simulink model "sscv_wind_turbine"  (R2024a)
settings: Solver=ode23t  StartTime=0.0  StopTime=simT  RelTol=1e-3  AbsTol=1e-3
PreLoadFcn:
  | sscv_wind_turbine_input
values from neighbouring files (symbols this model uses):
  actuatorRampRate = 20    [sscv_wind_turbine_input.m]
  brakePressure = 100    [sscv_wind_turbine_input.m]
  controllerTimeConstant = 2    [sscv_wind_turbine_input.m]
  Derating = [12 13 14 15 16 17 18 19 20 1 4 7 ... (18 elements, 9x2)]    [sscv_wind_turbine_Derating.mat]
  generatorEfficiency = 90    [sscv_wind_turbine_input.m]
  generatorLumpedInductance = 1.9160e-04    (= 0.0001916)    [sscv_wind_turbine_input.m]
  generatorLumpedResistance = 0.0027    [sscv_wind_turbine_input.m]
  gridFrequency = 60    [sscv_wind_turbine_input.m]
  iGenerationGain = 1    [sscv_wind_turbine_input.m]
  maxPitchAngle = max(pitch)    [sscv_wind_turbine_input.m]
  minPitchAngle = min(pitch)    [sscv_wind_turbine_input.m]
  mpptOmega = [502.335 613.965 753.5025 865.1325 1004.67 1116.3 1200.0225 1200.0225 1200.0225]    [sscv_wind_turbine_MPPT.mat]
  mpptPower = [0.0596400180021 0.116487570967 0.201285060757 0.319665137738 0.477120144017 0.679427108153 0.931130687114 1.22525336077 1.55330342875]    [sscv_wind_turbine_MPPT.mat]
  mpptWindSpeed = [4 5 6 7 8 9 10 11 12]    [sscv_wind_turbine_MPPT.mat]
  pGenerationGain = 0.1    [sscv_wind_turbine_input.m]
  pGeneratorBrakeLimit = 0.50    (= 0.5)    [sscv_wind_turbine_input.m]
  pitchBrakeAngle = 95    [sscv_wind_turbine_input.m]
  turbineRatedPower = 1.5    [sscv_wind_turbine_input.m]
  vWindRated = 12    [sscv_wind_turbine_input.m]
  wAtGeneratorRatedPower = wTurbineCutOut*gearRatio    (= 1227.93)    [sscv_wind_turbine_input.m]
  wGeneratorBrakeLimit = 0.50    (= 0.5)    [sscv_wind_turbine_input.m]
undefined symbols (not defined in the file or in its folder): ee_sli_rtmsupport, G, gcbh
libraries: fl_lib x18, simulink x15, nesl_utility x13, ee_lib x10, sdl_lib x6, eeGeneralControl x3, eeGeneralMeasurement x2
(part 1 of 2)
CloseFcn:
  | try,close(h_sscv_wind_turbine),end
  | clear h_sscv_wind_turbine
  | 
  | clear airDensity cp pitch TSR turbineRadius
  | clear vWindThreshold wThreshold vWindCutInLower
  | clear vWindCutOut vWindCutInUpper vWindRated
  | clear wTurbineCutIn wTurbineCutOut wTurbinePark
  | clear pitchBrakeAngle minPitchAngle maxPitchAngle
  | clear actuatorRampRate controllerTimeConstant
  | clear turbineRatedPower pGenerationGain
  | clear brakePressure brakeTorqueRadius
  | clear brakePistonArea brakeStaticFrictionCoeff
  | clear brakeKineticFrictionCoeff brakeClutchVelocityTol
  | clear brakeThresholdPressure numFrictionSurfaces
  | clear rotorBladeInertia generatorInertia
  | clear carrierShaftInertia stepShaftInertia
  | clear ringSunTeethRatio firstStepTeethRatio
  | clear secondStepTeethRatio windProfile
  | clear Derating gearRatio
  | clear generatorEfficiency mpptOmega mpptPower
  | clear generatorLumpedInductance generatorLumpedResistance
  | clear gridFrequency iGenerationGain
  | clear mpptWindSpeed transformerPrimaryVoltage
  | clear transformerRatedPower transformerSecondaryVoltage
  | clear wGeneratorBrakeLimit wAtGeneratorRatedPower
  | clear cpBraking simT pGeneratorBrakeLimit
  | clear windProfile1 windProfile2 windProfile3
  | clear numTSR
  | clear logsout_sscv_wind_turbine
  | clear simlog_sscv_wind_turbine
Description:
  | Wind Turbine
settings Model: Creator=The MathWorks, Inc.  LastModifiedBy=The MathWorks, Inc.
settings SolverCC: AutoScaleAbsTol=off  MaxConsecutiveMinStep=5  AlgebraicLoopSolver=TrustRegion  MaxZcPerStep=1
settings DataIOCC: SaveOutput=off  DSMLogging=off  SaveTime=off  ReturnWorkspaceOutputs=off  SignalLoggingName=logsout_sscv_wind_turbine
settings OptimizationCC: ReuseModelBlockBuffer=off
settings DebuggingCC: UnconnectedInputMsg=warning  UnconnectedOutputMsg=warning  UnconnectedLineMsg=warning
settings ModelReferenceCC: EnableRefExpFcnMdlSchedulingChecks=on
settings RTWCC: GPUComputeCapability=3.5  DLArmComputeVersion=19.05
settings SimscapeCC: SimscapeLogType=all  SimscapeLogSimulationStatistics=on  SimscapeLogName=simlog_sscv_wind_turbine  SimscapeLogDataHistory=10000000

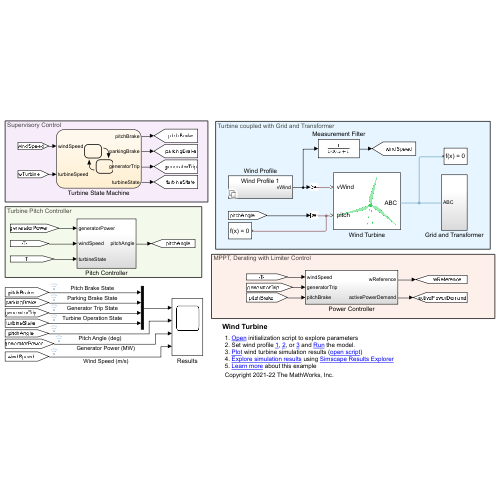
[thumbnail: Simulink's stored preview of the top-level diagram]
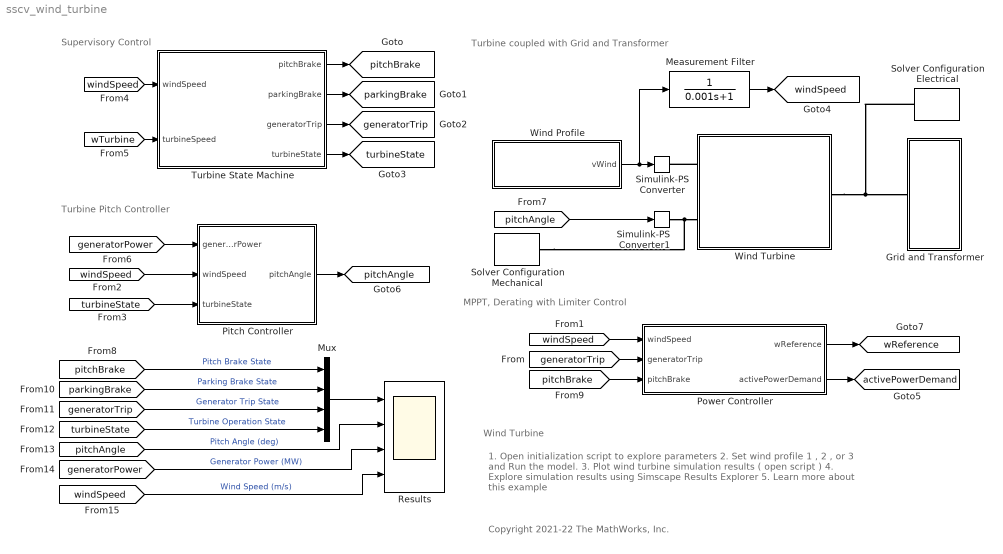
== system sscv_wind_turbine ==
  note: MPPT, Derating with Limiter Control
  note: Turbine coupled with Grid and Transformer
  note: Turbine Pitch Controller
  note: Supervisory Control
  note: 1. Open initialization script to explore parameters
      | 2. Set wind profile 1 , 2 , or 3 and Run the model.
      | 3. Plot wind turbine simulation results ( open script )
      | 4. Explore simulation results using Simscape Results Explorer
      | 5. Learn more about this example
  note: Wind Turbine
  note: Copyright 2021-22 The MathWorks, Inc.
  Grid and Transformer : Subsystem
  Measurement Filter : TransferFcn  Denominator=[0.001 1]
  Mux : Mux
  Pitch Controller : Subsystem
  Power Controller : Subsystem
  Results : Scope  NumInputPorts=4
  Simulink-PS Converter : nesl_utility/Simulink-PS Converter  PhysicalDomain=network_engine_domain  SubClassName=ps_input  LeftPortType=input  RightPortType=output  PseudoPeriodic=off  Frequencies=[]  NoiseDistribution=none  NoiseParameters=[]  Unit=m/s  AffineConversion=off  FilteringAndDerivatives=filter  SimscapeFilterOrder=1  InputFilterTimeConstant=0.001  UdotUserProvided=0
  Simulink-PS Converter1 : nesl_utility/Simulink-PS Converter  PhysicalDomain=network_engine_domain  SubClassName=ps_input  LeftPortType=input  RightPortType=output  PseudoPeriodic=off  Frequencies=[]  NoiseDistribution=none  NoiseParameters=[]  Unit=deg  AffineConversion=off  FilteringAndDerivatives=filter  SimscapeFilterOrder=1  InputFilterTimeConstant=0.001  UdotUserProvided=0
  Solver Configuration Electrical : nesl_utility/Solver Configuration  PhysicalDomain=network_engine_domain  SubClassName=solver  LeftPortType=input  RightPortType=generic  Tones=[]  Harmonics=[]  SimulateNoise=off  Profile=off  UseLocalSampling=off  EnableSwitchedLinearOptims=on  FrequencyDomain=off  UseCCode=off  RelTol=0.001  AbsTol=0.001  MinStep=1e-09  ToWorkspace=off  RevertToSquareIcSolve=off  NumHomotopyIterations=100  PhasorMode=off  PhasorModeNumHarmonics=1  ConsistencySolver=NEWTON_FTOL  IndexReductionMethod=DerivativeReplacement  DoDC=off  ResidualTolerance=1e-09  ConsistencyTolSource=GLOBAL  ConsistencyAbsTol=0.001  ConsistencyRelTol=0.001  ConsistencyTolFactor=0.001  UseLocalSolver=off  LocalSolverChoice=NE_TRAPEZOIDAL_ADVANCER  ResolveIndetEquations=on  FunctionEvalNumThread=1  LocalSolverSampleTime=1e-5  DoFixedCost=off  MaxNonlinIter=3  MaxModeIter=2  ComputeImpulses=off  ImpulseIterations=2  LinearAlgebra=auto  LinearAlgebraNumThread=0  EquationFormulation=NE_TIME_EF  DelaysMemoryBudget=1024  AutomaticFiltering=on  FilteringTimeConstant=0.001  PartitionStorageMethod=AS_NEEDED  PartitionMemoryBudget=1024  PartitionMethod=ROBUST  MultibodyUseLocalSolver=off  MultibodyLocalSolverChoice=ODE1  MultibodyLocalSolverSampleTime=0.001
  Solver Configuration Mechanical : nesl_utility/Solver Configuration  PhysicalDomain=network_engine_domain  SubClassName=solver  LeftPortType=input  RightPortType=generic  Tones=[]  Harmonics=[]  SimulateNoise=off  Profile=off  UseLocalSampling=off  EnableSwitchedLinearOptims=on  FrequencyDomain=off  UseCCode=off  RelTol=0.001  AbsTol=0.001  MinStep=1e-09  ToWorkspace=off  RevertToSquareIcSolve=off  NumHomotopyIterations=100  PhasorMode=off  PhasorModeNumHarmonics=1  ConsistencySolver=NEWTON_FTOL  IndexReductionMethod=DerivativeReplacement  DoDC=off  ResidualTolerance=1e-09  ConsistencyTolSource=GLOBAL  ConsistencyAbsTol=0.001  ConsistencyRelTol=0.001  ConsistencyTolFactor=0.001  UseLocalSolver=off  LocalSolverChoice=NE_TRAPEZOIDAL_ADVANCER  ResolveIndetEquations=on  FunctionEvalNumThread=1  LocalSolverSampleTime=0.001  DoFixedCost=off  MaxNonlinIter=3  MaxModeIter=2  ComputeImpulses=off  ImpulseIterations=2  LinearAlgebra=auto  LinearAlgebraNumThread=0  EquationFormulation=NE_TIME_EF  DelaysMemoryBudget=1024  AutomaticFiltering=on  FilteringTimeConstant=0.001  PartitionStorageMethod=AS_NEEDED  PartitionMemoryBudget=1024  PartitionMethod=ROBUST  MultibodyUseLocalSolver=off  MultibodyLocalSolverChoice=ODE1  MultibodyLocalSolverSampleTime=0.001
  Turbine State Machine : Stateflow chart  TreatAsAtomicUnit=on
  Wind Profile : Subsystem  Variant=on  VariantControl=Choice
  Wind Turbine : Subsystem
      mask Display:
      | image('sscv_wind_turbine.PNG');
      | port_label('LConn',1,' vWind')
      | port_label('LConn',2,' pitch')
      | port_label('RConn',1,'ABC ')
  tag scope: activePowerDemand=global, generatorTrip=global, parkingBrake=global, pitchAngle=global, pitchBrake=global, turbineState=global, wReference=global, windSpeed=global
  wires:
  Turbine State Machine/1(pitchBrake) -> [pitchBrake]
  Turbine State Machine/2(parkingBrake) -> [parkingBrake]
  Turbine State Machine/3(generatorTrip) -> [generatorTrip]
  Turbine State Machine/4(turbineState) -> [turbineState]
  [windSpeed] -> Turbine State Machine/1(windSpeed)
  [wTurbine] -> Turbine State Machine/2(turbineSpeed)
  [generatorPower] -> Pitch Controller/1(generatorPower)
  [turbineState] -> Pitch Controller/3(turbineState)
  [pitchAngle] -> Simulink-PS Converter1/1
  Measurement Filter/1 -> [windSpeed]
  [windSpeed] -> Power Controller/1(windSpeed)
  Power Controller/1(wReference) -> [wReference]
  Power Controller/2(activePowerDemand) -> [activePowerDemand]
  [generatorTrip] -> Power Controller/2(generatorTrip)
  Pitch Controller/1(pitchAngle) -> [pitchAngle]
  [windSpeed] -> Pitch Controller/2(windSpeed)
  [pitchBrake] -> Power Controller/3(pitchBrake)
  [pitchBrake] -> Mux/1  "Pitch Brake State"
  [parkingBrake] -> Mux/2  "Parking Brake State"
  [generatorTrip] -> Mux/3  "Generator Trip State"
  [turbineState] -> Mux/4  "Turbine Operation State"
  Mux/1 -> Results/1
  [pitchAngle] -> Results/2  "Pitch Angle (deg)"
  [generatorPower] -> Results/3  "Generator Power (MW)"
  [windSpeed] -> Results/4  "Wind Speed (m/s)"
  Wind Profile/1(vWind) -> Measurement Filter/1, Simulink-PS Converter/1
  connections:
  Wind Turbine/RConn1 -- Solver Configuration Electrical/RConn1 -- Grid and Transformer/LConn1
  Simulink-PS Converter1/RConn1 -- Solver Configuration Mechanical/RConn1 -- Wind Turbine/LConn2
  Wind Turbine/LConn1 -- Simulink-PS Converter/RConn1

== system sscv_wind_turbine/Grid and Transformer ==
  Electrical Reference : fl_lib/Electrical/Electrical Elements/Electrical Reference
  Grid : ee_lib/Sources/Voltage Source (Three-Phase)  vline_rms=transformerPrimaryVoltage kV  shift=0 deg  freq=gridFrequency Hz  impedance_option=0  SShortCircuit=1e6 A*V  XR=15  R=0.01 Ohm  L=3.97e-4 H  harmonic_option=0  harmonic_orders=[5, 7, 11, 13]  harmonic_ratios=[.1, .1, .1, .1]  G_parasitic=0 1/Ohm  I_specify=off  I_priority=None  I=[0, 0, 0] A  I_nominal_specify=off  I_nominal_value=1  I_nominal_unit=A
  Neutral Port (Three-Phase) : ee_lib/Connectors & References/Neutral Port (Three-Phase)  G_parasitic=1e-12 1/Ohm
      settings: InternalSimscapePortConfiguration="{\"Bottom\":[],\"Left\":[{\"id\":\"N\",\"label\":\"~\",\"type\":\"foundation.electrical.three_phase\"}],\"Right\":[{\"id\":\"n\",\"label\":\"n\",\"type\":\"foundation.electrical.electrical\"}],\"Top\":[]}"
  Parasitic Conductance : ee_lib/Passive/RLC Assemblies/RLC (Three-Phase)  component_structure=ee.enum.rlc.structure.R  R=100000 Ohm  L=1e-3 H  C=1e-6 F  R_parasitic=0 Ohm  G_parasitic=0 1/Ohm  IL_specify=off  IL_priority=High  IL=[0, 0, 0] A  IL_nominal_specify=off  IL_nominal_value=1  IL_nominal_unit=A  VC_specify=off  VC_priority=High  VC=[0, 0, 0] V  VC_nominal_specify=off  VC_nominal_value=1  VC_nominal_unit=V
      settings: InternalSimscapePortConfiguration="{\"Bottom\":[],\"Left\":[{\"id\":\"N1\",\"label\":\"~1\",\"type\":\"foundation.electrical.three_phase\"}],\"Right\":[{\"id\":\"N2\",\"label\":\"~2\",\"type\":\"foundation.electrical.three_phase\"}],\"Top\":[]}"
  Transformer : ee_lib/Passive/Transformers/Two-Winding Transformer (Three-Phase)  SRated=transformerRatedPower MW  FRated=gridFrequency Hz  Winding1Connection=ee.enum.windingconnection.Y  VRated1=transformerPrimaryVoltage kV  Winding2Connection=ee.enum.windingconnection.Y  VRated2=transformerSecondaryVoltage kV  CoreType=ee.enum.coretype.threelimb  pu_Rw1=0.0001  pu_Rw2=0.0001  leakage_reactance_option=ee.enum.transformer_leakage.exclude  pu_Xl1=0.05  pu_Xl2=0.05  magnetizing_resistance_option=ee.enum.transformer_magnetizingResistance.exclude  pu_Rm=500  magnetizing_reactance_option=ee.enum.transformer_magnetizingReactance.exclude  saturation_option=ee.enum.transformer_saturation.exclude  pu_Xm=500  current_data=[0, .002, 1, 2]  magnetic_flux_data=[0, 1.2, 1.5, 1.51]  pu_X0=0.5  i1_specify=off  i1_priority=None  i1=[0, 0, 0] A  i1_nominal_specify=off  i1_nominal_value=1  i1_nominal_unit=A  i2_specify=off  i2_priority=None  i2=[0, 0, 0] A  i2_nominal_specify=off  i2_nominal_value=1  i2_nominal_unit=A  phi_specify=off  phi_priority=None  phi=[0, 0, 0]  phi_nominal_specify=off  phi_nominal_value=1  phi_nominal_unit=1  power_dissipated_specify=off  power_dissipated_priority=None  power_dissipated=0 W  power_dissipated_nominal_specify=off  power_dissipated_nominal_value=1  power_dissipated_nominal_unit=W
      settings: InternalSimscapePortConfiguration="{\"Bottom\":[],\"Left\":[{\"id\":\"N1\",\"label\":\"~1\",\"type\":\"foundation.electrical.three_phase\"}],\"Right\":[{\"id\":\"N2\",\"label\":\"~2\",\"type\":\"foundation.electrical.three_phase\"}],\"Top\":[]}"
  ABC : PMIOPort  Side=Left
  connections:
  Transformer/RConn1 -- Parasitic Conductance/LConn1 -- ABC/RConn1
  Neutral Port (Three-Phase)/RConn1 -- Electrical Reference/LConn1 -- Grid/LConn1
  Neutral Port (Three-Phase)/LConn1 -- Parasitic Conductance/RConn1
  Transformer/LConn1 -- Grid/RConn1

== system sscv_wind_turbine/Pitch Controller ==
  generatorPower : Inport
  windSpeed : Inport  Port=2
  turbineState : Inport  Port=3
  Merge : Merge  Inputs=3
  Pitch Change Rate Limiter : RateLimiter  RisingSlewLimit=actuatorRampRate  FallingSlewLimit=-actuatorRampRate  SampleTimeMode=inherited
  Transfer Fcn1 : TransferFcn  Denominator=[1e-4 1]
  "Turbine State 0 : Park Brake and Turbine State 3 : Pitch Brake" : Subsystem
      settings: PortSchema="{\"entries\":[{\"content\":{\"sides\":[{\"content\":{\"connectorIds\":[\"In1\"]},\"type\":\"ConnectorPlacement.EquallySpacedRectSide\",\"uuid\":\"c81c0fc4-0b31-4a43-acf3-ef02f67f12ef\"},{\"content\":{\"connectorIds\":[\"In2\",\"Out1\"],\"side\":\"RIGHT\"},\"type\":\"ConnectorPlacement.EquallySpacedRectSide\",\"uuid\":\"c20c9bc8-a4c7-4c6f-a8fa-fe8ff88298f7\"},{\"content\":{\"connectorIds\":[],\"side\":\"TOP\"},\"type\":\"ConnectorPlacement.EquallySpacedRectSide\",\"uuid\":\"2b845051-401f-423c-a453-0a1243a015d1\"}]},\"type\":\"ConnectorPlacement.EquallySpacedConnector\",\"uuid\":\"502647d6-ee95-4637-92b5-6d3c38784edf\"}],\"packageUris\":[\"http://schema.mathworks.com/mf0/Connector/R2020b\"],\"version\":\"1.0\"}"
  "Turbine State 1 : Startup Condition" : Subsystem
  "Turbine State 2 : Power Generation Condition" : Subsystem
  pitchAngle : Outport
  wires:
  Pitch Change Rate Limiter/1 -> pitchAngle/1
  turbineState/1 -> "Turbine State 2 : Power Generation Condition"/3(turbineState), "Turbine State 0 : Park Brake and Turbine State 3 : Pitch Brake"/1(turbineState), "Turbine State 1 : Startup Condition"/1(turbineState)
  generatorPower/1 -> "Turbine State 2 : Power Generation Condition"/1(generatorPower)
  Merge/1 -> Pitch Change Rate Limiter/1, Transfer Fcn1/1
  "Turbine State 0 : Park Brake and Turbine State 3 : Pitch Brake"/1(pitchAngle) -> Merge/1
  "Turbine State 1 : Startup Condition"/1(pitchAngle) -> Merge/2
  "Turbine State 2 : Power Generation Condition"/1(pitchAngle) -> Merge/3
  windSpeed/1 -> "Turbine State 2 : Power Generation Condition"/2(windSpeed)
  Transfer Fcn1/1 -> "Turbine State 0 : Park Brake and Turbine State 3 : Pitch Brake"/2(pitchState)

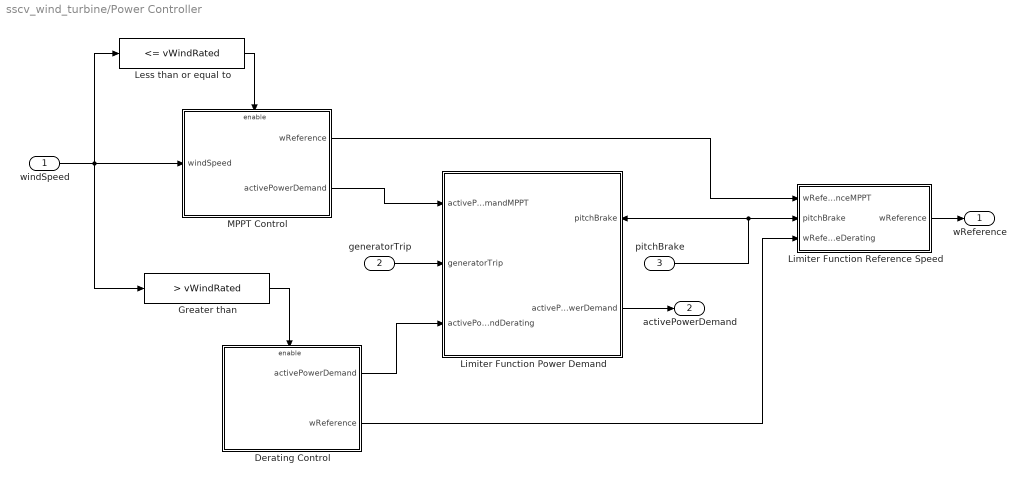
== system sscv_wind_turbine/Power Controller ==
  windSpeed : Inport
  generatorTrip : Inport  Port=2
  pitchBrake : Inport  Port=3
  Derating Control : Subsystem
  Greater than : simulink/Logic and Bit Operations/Compare To Constant  relop=>  const=vWindRated  OutDataTypeStr=boolean
  Less than or equal to : simulink/Logic and Bit Operations/Compare To Constant  relop=<=  const=vWindRated  OutDataTypeStr=boolean
  Limiter Function Power Demand : Subsystem
      settings: PortSchema="{\"entries\":[{\"content\":{\"sides\":[{\"content\":{\"connectorIds\":[\"In1\",\"In2\",\"In3\"]},\"type\":\"ConnectorPlacement.EquallySpacedRectSide\",\"uuid\":\"b03cf57d-370b-4fa1-bd93-9b836e03697e\"},{\"content\":{\"connectorIds\":[\"In4\",\"Out1\"],\"side\":\"RIGHT\"},\"type\":\"ConnectorPlacement.EquallySpacedRectSide\",\"uuid\":\"152758c3-43df-447a-a50f-afca466b3eeb\"},{\"content\":{\"connectorIds\":[],\"side\":\"TOP\"},\"type\":\"ConnectorPlacement.EquallySpacedRectSide\",\"uuid\":\"d053be3f-8f1f-4fa1-8d53-3d41a1fdecc7\"}]},\"type\":\"ConnectorPlacement.EquallySpacedConnector\",\"uuid\":\"ad588a80-a06e-49b6-a4d2-a4be271ff49a\"}],\"packageUris\":[\"http://schema.mathworks.com/mf0/Connector/R2020b\"],\"version\":\"1.0\"}"
  Limiter Function Reference Speed : Subsystem
  MPPT Control : Subsystem
  wReference : Outport
  activePowerDemand : Outport  Port=2
  wires:
  windSpeed/1 -> Greater than/1, Less than or equal to/1, MPPT Control/1(windSpeed)
  Less than or equal to/1 -> MPPT Control/Enable
  Greater than/1 -> Derating Control/Enable
  MPPT Control/2(activePowerDemand) -> Limiter Function Power Demand/1(activePowerDemandMPPT)
  generatorTrip/1 -> Limiter Function Power Demand/2(generatorTrip)
  Derating Control/1(activePowerDemand) -> Limiter Function Power Demand/3(activePowerDemandDerating)
  Limiter Function Power Demand/1(activePowerDemand) -> activePowerDemand/1
  pitchBrake/1 -> Limiter Function Reference Speed/2(pitchBrake), Limiter Function Power Demand/4(pitchBrake)
  MPPT Control/1(wReference) -> Limiter Function Reference Speed/1(wReferenceMPPT)
  Derating Control/2(wReference) -> Limiter Function Reference Speed/3(wReferenceDerating)
  Limiter Function Reference Speed/1(wReference) -> wReference/1

== system sscv_wind_turbine/Wind Profile ==
  Wind Profile 1 : Subsystem  VariantControl=windProfile1
  Wind Profile 2 : Subsystem  VariantControl=windProfile2
  Wind Profile 3 : Subsystem  VariantControl=windProfile3
  vWind : Outport

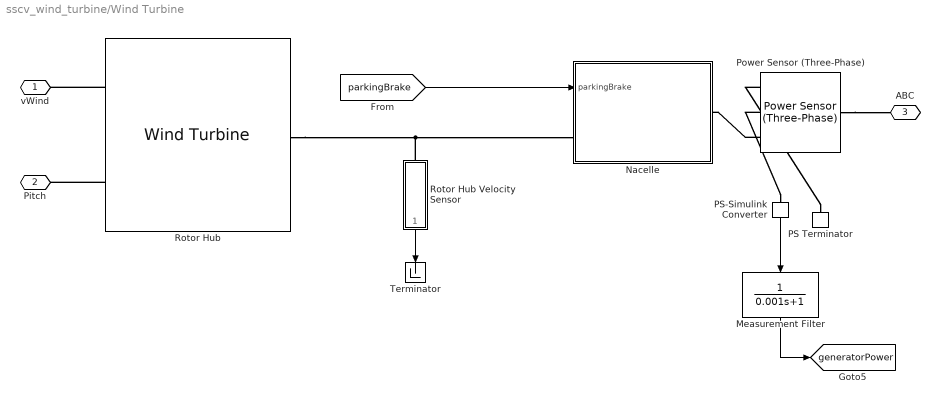
== system sscv_wind_turbine/Wind Turbine ==
  Measurement Filter : TransferFcn  Denominator=[0.001 1]
  Nacelle : Subsystem
  PS Terminator : fl_lib/Physical Signals/Sinks/PS Terminator
  PS-Simulink Converter : nesl_utility/PS-Simulink Converter  PhysicalDomain=network_engine_domain  SubClassName=ps_output  LeftPortType=input  RightPortType=output  PseudoPeriodic=off  Frequencies=[]  VectorFormat=inherit  Unit=MW  AffineConversion=off
  Power Sensor (Three-Phase) : ee_lib/Sensors & Transducers/Power Sensor (Three-Phase)  load_type=ee.enum.passive.type_balanced.balanced  f0=60 Hz  config=ee.enum.with_neutral.no  rho=1
      settings: InternalSimscapePortConfiguration="{\"Bottom\":[],\"Left\":[{\"id\":\"N1\",\"label\":\"~1\",\"type\":\"foundation.electrical.three_phase\"}],\"Right\":[{\"id\":\"N2\",\"label\":\"~2\",\"type\":\"foundation.electrical.three_phase\"}],\"Top\":[{\"id\":\"Pm\",\"label\":\"P\",\"type\":\"output\"},{\"id\":\"Qm\",\"label\":\"Q\",\"type\":\"output\"}]}"
  Rotor Hub : sdl_lib/Engines & Motors/Wind Turbine  parameterization=sdl.enum.WindTurbineParameterization.PowerThrust  R_rotor=turbineRadius m  pitch_TLU=pitch deg  lambda_TLU=TSR  Cp_TLU=cp  Ct_TLU=[0.0777, 0.1421, 0.3753, 0.6599, 0.8160, 0.9112, 0.9925, 1.0708, 1.1147; 0.0762, 0.1377, 0.3570, 0.5529, 0.6291, 0.6573, 0.6706, 0.6421, 0.6284; 0.0682, 0.1292, 0.3362, 0.4664, 0.4874, 0.4547, 0.3915, 0.2865, 0.2249; -0.05 * ones(1, 9)]  n_blades=3  radial_TLU=[.1, .17, .23, .36, .5, .63, 1]  twist_TLU=[13.31, 13.31, 11.48, 9.01, 6.54, 4.19, .11] deg  chord_TLU=[.068, .074, .076, .069, .061, .053, .023]  alpha_TLU=[-180 : 10 : 180] deg  Cl_TLU=[0, 0, 0, 0, 0, 0, 0; 0, .397, .547, .547, .735, .788, .749; 0, .642, .685, .685, .695, .67, .659; 0, .757, .816, .816, .828, .797, .783; 0, .762, .832, .832, .846, .813, .798; 0, .68, .756, .756, .771, .739, .724; 0, .532, .609, .609, .624, .596, .581; 0, .337, .411, .411, .426, .403, .39; 0, .114, .182, .182, .195, .179, .169; 0, -.12, -.061, -.061, -.05, -.06, -.067; 0, -.349, -.302, -.302, -.294, -.295, -.299; 0, -.557, -.523, -.523, -.518, -.512, -.512; 0, -.727, -.708, -.708, -.706, -.693, -.689; 0, -.842, -.838, -.838, -.839, -.82, -.814; 0, -.886, -.895, -.895, -.898, -.875, -.866; 0, -.839, -.858, -.858, -.862, -.838, -.829; 0, -.685, -1.013, -1.013, -.815, -.869, -.958; 0, -.311, -.8496, -.8496, -.8284, -.8284, -.711; 0, .137, .288, .288, .444, .521, .442; 0, 1.368, 1.458, 1.458, 1.442, 1.358, 1.382; 0, 1.7825, 1.398, 1.398, 1.354, 1.311, 1.428; 0, 1.904, 1.265, 1.265, 1.076, .962, .926; 0, 1.903, 1.258, 1.258, 1.064, .95, .804; 0, 1.69, 1.146, 1.146, .98, .884, .763; 0, 1.323, .932, .932, .81, .74, .656; 0, .88, .657, .657, .582, .54, .495; 0, .449, .362, .362, .326, .304, .291; 0, .124, .092, .092, .072, .053, .053; 0, -.118, -.15, -.15, -.17, -.198, -.199; 0, -.348, -.379, -.379, -.399, -.434, -.436; 0, -.549, -.578, -.578, -.596, -.637, -.64; 0, -.702, -.727, -.727, -.743, -.787, -.79; 0, -.787, -.807, -.807, -.821, -.864, -.868; 0, -.782, -.797, -.797, -.806, -.847, -.85; 0, -.664, -.673, -.673, -.679, -.711, -.714; 0, -.41, -.547, -.547, -.735, -.788, -.749; 0, 0, 0, 0, 0, 0, 0]  Cd_TLU=[.35, .0602, .0267, .0267, .0202, .0185, .0198; .35, .1107, .0968, .0968, .0943, .0945, .0955; .35, .3045, .2876, .2876, .2848, .2809, .2807; .35, .5355, .5232, .5232, .5215, .5112, .5086; .35, .7685, .7656, .7656, .766, .7485, .7427; .35, .9788, .9882, .9882, .9911, .9665, .9574; .35, 1.1499, 1.173, 1.173, 1.1787, 1.1476, 1.1355; .35, 1.2716, 1.3084, 1.3084, 1.3168, 1.2805, 1.2656; .35, 1.3378, 1.3875, 1.3875, 1.3984, 1.3582, 1.341; .35, 1.346, 1.407, 1.407, 1.4201, 1.3774, 1.3587; .35, 1.2964, 1.3664, 1.3664, 1.3811, 1.3376, 1.3181; .35, 1.1918, 1.2676, 1.2676, 1.2833, 1.2409, 1.2212; .35, 1.0376, 1.1156, 1.1156, 1.1315, 1.0919, 1.0731; .35, .8429, .9187, .9187, .9341, .899, .882; .35, .6215, .6904, .6904, .7042, .6754, .661; .35, .3932, .4503, .4503, .4616, .4405, .4295; .35, .1861, .2388, .2388, .2237, .1983, .1785; .35, .0931, .0718, .0718, .0287, .0287, .0111; .35, .0113, .0087, .0087, .0065, .0057, .0052; .35, .0393, .0192, .0192, .0262, .0255, .015; .35, .3998, .2689, .2689, .228, .1987, .2379; .35, .8441, .5843, .5843, .5149, .4813, .4294; .35, 1.2873, .897, .897, .7901, .7396, .6452; .35, 1.6401, 1.1686, 1.1686, 1.0378, .9781, .8664; .35, 1.836, 1.3647, 1.3647, 1.2333, 1.1796, 1.0693; .35, 1.8347, 1.4621, 1.4621, 1.3587, 1.3297, 1.2438; .35, 1.6334, 1.4544, 1.4544, 1.4063, 1.4202, 1.3809; .35, 1.3879, 1.3938, 1.3938, 1.3985, 1.4512, 1.4565; .35, 1.3795, 1.3798, 1.3798, 1.381, 1.4294, 1.4345; .35, 1.3114, 1.3063, 1.3063, 1.3041, 1.3464, 1.3512; .35, 1.1864, 1.1763, 1.1763, 1.1709, 1.2057, 1.2099; .35, 1.0102, .9962, .9962, .9883, 1.0144, 1.0179; .35, .7935, .7771, .7771, .7676, .7845, .7871; .35, .5532, .5364, .5364, .5264, .5346, .5363; .35, .3147, .3, .3, .2912, .2922, .2931; .35, .1144, .1051, .1051, .0995, .0969, .0971; .35, .0602, .0267, .0267, .0202, .0185, .0198]  n_blade_discretization=20  model_thrust=false  model_inertia=sdl.enum.model_inertia.on  rotor_inertia=rotorBladeInertia kg*m^2  init_rot_vel=0 rad/s  rho_air=airDensity kg/m^3  v_thr=0.01 m/s  w_thr=0.01 rad/s  root_pitch=0 deg  expose_port_C=0
      settings: InternalSimscapePortConfiguration="{\"Bottom\":[],\"Left\":[{\"id\":\"vWind\",\"label\":\"V\",\"type\":\"input\"},{\"id\":\"pitch\",\"label\":\"β\",\"type\":\"input\"}],\"Right\":[{\"id\":\"R\",\"label\":\"R\",\"type\":\"foundation.mechanical.rotational.rotational\"}],\"Top\":[]}"
  Rotor Hub Velocity Sensor : Subsystem
  Terminator : Terminator
  vWind : PMIOPort  Side=Left
  Pitch : PMIOPort  Port=2  Side=Left
  ABC : PMIOPort  Port=3  Side=Right
  tag scope: generatorPower=global
  wires:
  Rotor Hub Velocity Sensor/1(wTurbine) -> Terminator/1
  [parkingBrake] -> Nacelle/1(parkingBrake)
  PS-Simulink Converter/1 -> Measurement Filter/1
  Measurement Filter/1 -> [generatorPower]
  connections:
  Rotor Hub/LConn1 -- vWind/RConn1
  Rotor Hub/LConn2 -- Pitch/RConn1
  Rotor Hub Velocity Sensor/LConn1 -- Rotor Hub/RConn1 -- Nacelle/LConn1
  Power Sensor (Three-Phase)/RConn1 -- ABC/RConn1
  Power Sensor (Three-Phase)/LConn1 -- Nacelle/RConn1
  Power Sensor (Three-Phase)/LConn2 -- PS-Simulink Converter/LConn1
  Power Sensor (Three-Phase)/LConn3 -- PS Terminator/LConn1

== system sscv_wind_turbine/Pitch Controller/Turbine State 0 : Park Brake and Turbine State 3 : Pitch Brake ==
  turbineState : Inport
  pitchState : Inport  Port=2
  Compare To Constant : simulink/Logic and Bit Operations/Compare To Constant  relop===  const=0  OutDataTypeStr=boolean
  Compare To Constant1 : simulink/Logic and Bit Operations/Compare To Constant  relop===  const=3  OutDataTypeStr=boolean
  OR : Logic  Operator=OR  IconShape=distinctive  AllPortsSameDT=off  OutDataTypeStr=boolean
  Turbine State 0 an 3 : Subsystem
  pitchAngle : Outport
  wires:
  Turbine State 0 an 3/1(pitchAngle) -> pitchAngle/1
  turbineState/1 -> Compare To Constant1/1, Compare To Constant/1
  pitchState/1 -> Turbine State 0 an 3/1(pitchState)
  OR/1 -> Turbine State 0 an 3/Enable
  Compare To Constant/1 -> OR/1
  Compare To Constant1/1 -> OR/2

== system sscv_wind_turbine/Pitch Controller/Turbine State 1 : Startup Condition ==
  turbineState : Inport
  Compare To Constant : simulink/Logic and Bit Operations/Compare To Constant  relop===  const=1  OutDataTypeStr=boolean
  Turbine State 1 : Subsystem
  pitchAngle : Outport
  wires:
  turbineState/1 -> Compare To Constant/1
  Compare To Constant/1 -> Turbine State 1/Enable
  Turbine State 1/1(pitchAngle) -> pitchAngle/1

== system sscv_wind_turbine/Pitch Controller/Turbine State 2 : Power Generation Condition ==
  generatorPower : Inport
  windSpeed : Inport  Port=2
  turbineState : Inport  Port=3
  Compare To Constant : simulink/Logic and Bit Operations/Compare To Constant  relop===  const=2  OutDataTypeStr=boolean
  Turbine State 2 : Subsystem
  pitchAngle : Outport
  wires:
  Turbine State 2/1(pitchAngle) -> pitchAngle/1
  Compare To Constant/1 -> Turbine State 2/Enable
  turbineState/1 -> Compare To Constant/1
  generatorPower/1 -> Turbine State 2/1(generatorPower)
  windSpeed/1 -> Turbine State 2/2(windSpeed)

== system sscv_wind_turbine/Power Controller/Derating Control ==
  Enable : EnablePort  StatesWhenEnabling=reset
  Constant : Constant  Value=turbineRatedPower
  Constant1 : Constant  Value=wAtGeneratorRatedPower
  Gain : Gain  Gain=100/generatorEfficiency
  MW to W : Gain  Gain=1e6
  activePowerDemand : Outport
  wReference : Outport  Port=2
  wires:
  Constant1/1 -> wReference/1
  MW to W/1 -> activePowerDemand/1
  Constant/1 -> Gain/1
  Gain/1 -> MW to W/1

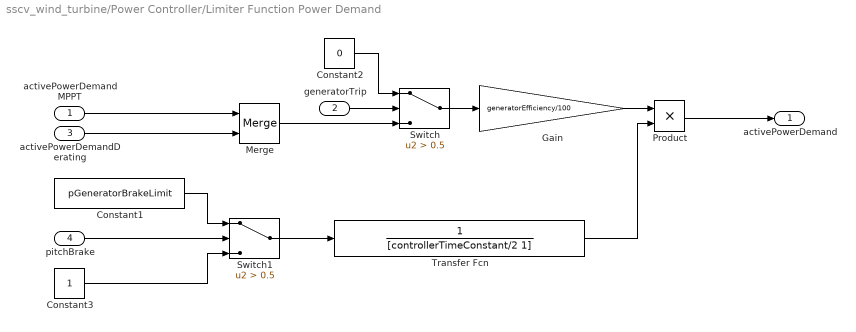
== system sscv_wind_turbine/Power Controller/Limiter Function Power Demand ==
  activePowerDemandMPPT : Inport
  generatorTrip : Inport  Port=2
  activePowerDemandDerating : Inport  Port=3
  pitchBrake : Inport  Port=4
  Constant1 : Constant  Value=pGeneratorBrakeLimit
  Constant2 : Constant  Value=0
  Constant3 : Constant
  Gain : Gain  Gain=generatorEfficiency/100
  Merge : Merge
  Product : Product
  Switch : Switch  Criteria=u2 > Threshold  Threshold=0.5  SaturateOnIntegerOverflow=off  InputSameDT=off
  Switch1 : Switch  Criteria=u2 > Threshold  Threshold=0.5  SaturateOnIntegerOverflow=off  InputSameDT=off
  Transfer Fcn : TransferFcn  Denominator=[controllerTimeConstant/2 1]
  activePowerDemand : Outport
  wires:
  generatorTrip/1 -> Switch/2
  Switch/1 -> Gain/1
  Constant2/1 -> Switch/1
  Merge/1 -> Switch/3
  activePowerDemandMPPT/1 -> Merge/1
  activePowerDemandDerating/1 -> Merge/2
  pitchBrake/1 -> Switch1/2
  Constant3/1 -> Switch1/3
  Constant1/1 -> Switch1/1
  Gain/1 -> Product/1
  Switch1/1 -> Transfer Fcn/1
  Product/1 -> activePowerDemand/1
  Transfer Fcn/1 -> Product/2

== system sscv_wind_turbine/Power Controller/Limiter Function Reference Speed ==
  wReferenceMPPT : Inport
  pitchBrake : Inport  Port=2
  wReferenceDerating : Inport  Port=3
  Constant : Constant
  Constant1 : Constant  Value=wGeneratorBrakeLimit
  Merge1 : Merge
  Product : Product
  Switch1 : Switch  Criteria=u2 > Threshold  Threshold=0.5  SaturateOnIntegerOverflow=off  InputSameDT=off
  Transfer Fcn : TransferFcn  Denominator=[controllerTimeConstant/2 1]
  wReference : Outport
  wires:
  pitchBrake/1 -> Switch1/2
  Constant1/1 -> Switch1/1
  wReferenceMPPT/1 -> Merge1/1
  wReferenceDerating/1 -> Merge1/2
  Merge1/1 -> Product/2
  Constant/1 -> Switch1/3
  Product/1 -> wReference/1
  Transfer Fcn/1 -> Product/1
  Switch1/1 -> Transfer Fcn/1

== system sscv_wind_turbine/Power Controller/MPPT Control ==
  windSpeed : Inport
  Enable : EnablePort  StatesWhenEnabling=reset
  MW to W : Gain  Gain=1e6
  mpptActivePowerDemand : Lookup_n-D  NumberOfTableDimensions=1  BreakpointsForDimension1=mpptWindSpeed  Table=mpptPower  InternalRulePriority=Speed  RndMeth=Simplest
  mpptOmega : Lookup_n-D  NumberOfTableDimensions=1  BreakpointsForDimension1=mpptWindSpeed  Table=mpptOmega  InternalRulePriority=Speed  RndMeth=Simplest
  wReference : Outport
  activePowerDemand : Outport  Port=2
  wires:
  mpptActivePowerDemand/1 -> MW to W/1
  mpptOmega/1 -> wReference/1
  windSpeed/1 -> mpptActivePowerDemand/1, mpptOmega/1
  MW to W/1 -> activePowerDemand/1

== system sscv_wind_turbine/Wind Profile/Wind Profile 1 ==
  Ramp : simulink/Sources/Ramp  slope=1  start=45  InitialOutput=15
  Saturation : Saturate  UpperLimit=22  LowerLimit=0
  vWind : Outport
  wires:
  Ramp/1 -> Saturation/1
  Saturation/1 -> vWind/1

== system sscv_wind_turbine/Wind Profile/Wind Profile 2 ==
  Add : Sum  Inputs=+
  Mux : Mux  Inputs=3
  Ramp : simulink/Sources/Ramp  slope=0.7  start=0  InitialOutput=0
  Ramp1 : simulink/Sources/Ramp  slope=0.7  start=115  InitialOutput=0
  Ramp2 : simulink/Sources/Ramp  slope=-0.7  start=160  InitialOutput=0
  Saturation : Saturate  UpperLimit=10  LowerLimit=0
  Saturation1 : Saturate  UpperLimit=12  LowerLimit=0
  Saturation2 : Saturate  UpperLimit=0  LowerLimit=-7
  vWind : Outport
  wires:
  Saturation1/1 -> Mux/2
  Ramp/1 -> Saturation/1
  Ramp2/1 -> Saturation2/1
  Add/1 -> vWind/1
  Saturation/1 -> Mux/1
  Ramp1/1 -> Saturation1/1
  Mux/1 -> Add/1
  Saturation2/1 -> Mux/3

== system sscv_wind_turbine/Wind Profile/Wind Profile 3 ==
  Ramp : simulink/Sources/Ramp  slope=1  start=45  InitialOutput=15
  Saturation : Saturate  UpperLimit=17  LowerLimit=0
  vWind : Outport
  wires:
  Ramp/1 -> Saturation/1
  Saturation/1 -> vWind/1

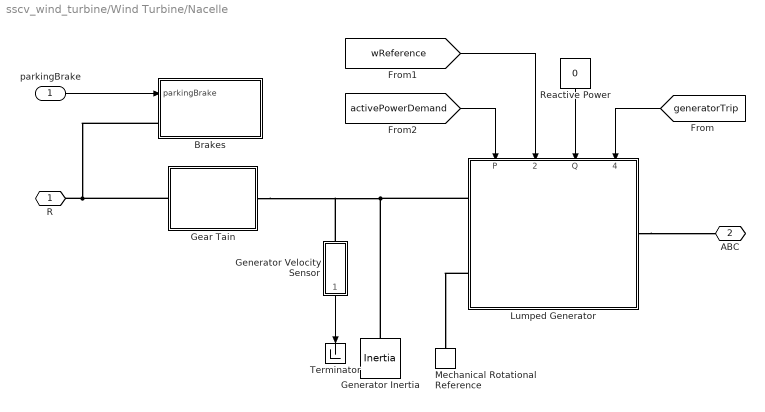
== system sscv_wind_turbine/Wind Turbine/Nacelle ==
  parkingBrake : Inport
  Brakes : Subsystem
  Gear Tain : Subsystem
  Generator Inertia : fl_lib/Mechanical/Rotational Elements/Inertia  inertia=generatorInertia kg*m^2  num_ports=foundation.enum.numPorts2.one  w_specify=on  w_priority=None  w=0 rad/s  w_nominal_specify=off  w_nominal_value=1  w_nominal_unit=rad/s  t_specify=off  t_priority=None  t=0 N*m  t_nominal_specify=off  t_nominal_value=1  t_nominal_unit=N*m
  "Generator Velocity Sensor " : Subsystem
  Lumped Generator : Subsystem  mask{ratedPower=turbineRatedPower, gridFreq=gridFrequency, genResistor=generatorLumpedResistance, genInductance=generatorLumpedInductance, genEfficiency=generatorEfficiency, ratedSpeed=wAtGeneratorRatedPower}
      mask prompts: ratedPower "Rated power (MW)"; gridFreq "Grid frequency (Hz)"; genResistor "Electrical generator lumped resistance (Ohm)"; genInductance "Electrical generator lumped leakage inductance (H)"; genEfficiency "Electrical generator effficiency"; ratedSpeed "Wind turbine speed at rated wind speed (rpm)"
      settings: PortSchema="{\"entries\":[{\"content\":{\"sides\":[{\"content\":{\"connectorIds\":[\"LConn1\",\"LConn2\"]},\"type\":\"ConnectorPlacement.EquallySpacedRectSide\",\"uuid\":\"600b86f2-4f8f-493b-ad26-1faa8bb85470\"},{\"content\":{\"connectorIds\":[\"RConn1\"],\"side\":\"RIGHT\"},\"type\":\"ConnectorPlacement.EquallySpacedRectSide\",\"uuid\":\"9e1649b7-9973-42e8-ab8f-93eff55c3d74\"},{\"content\":{\"connectorIds\":[\"In1\",\"In2\",\"In3\",\"In4\"],\"side\":\"TOP\"},\"type\":\"ConnectorPlacement.EquallySpacedRectSide\",\"uuid\":\"66dc1112-3744-4fa2-a344-a6dc92e314fc\"},{\"content\":{\"connectorIds\":[],\"side\":\"BOTTOM\"},\"type\":\"ConnectorPlacement.EquallySpacedRectSide\",\"uuid\":\"0ba4da35-be81-423d-9ede-c806323f0c4b\"}]},\"type\":\"ConnectorPlacement.EquallySpacedConnector\",\"uuid\":\"3b2d2e6e-f4ee-4b4b-84c0-3ef19b29de27\"}],\"packageUris\":[\"http://schema.mathworks.com/mf0/Connector/R2020b\"],\"version\":\"1.0\"}"
      mask Display: disp('Lumped Generator');
  Mechanical Rotational Reference : fl_lib/Mechanical/Rotational Elements/Mechanical Rotational Reference
  Reactive Power : Constant  Value=0
  Terminator : Terminator
  R : PMIOPort  Side=Left
  ABC : PMIOPort  Port=2  Side=Right
  wires:
  "Generator Velocity Sensor "/1(wGen) -> Terminator/1
  parkingBrake/1 -> Brakes/1(parkingBrake)
  [wReference] -> Lumped Generator/2(rotorSpeed)
  Reactive Power/1 -> Lumped Generator/3(Q)
  [activePowerDemand] -> Lumped Generator/1(P)
  [generatorTrip] -> Lumped Generator/4(generatorTrip)
  connections:
  Lumped Generator/LConn2 -- Mechanical Rotational Reference/LConn1
  Gear Tain/LConn1 -- Brakes/LConn1 -- R/RConn1
  Generator Inertia/LConn1 -- Lumped Generator/LConn1 -- Gear Tain/RConn1 -- "Generator Velocity Sensor "/LConn1
  Lumped Generator/RConn1 -- ABC/RConn1

== system sscv_wind_turbine/Wind Turbine/Rotor Hub Velocity Sensor ==
  Ideal Rotational Motion Sensor : fl_lib/Mechanical/Mechanical Sensors/Ideal Rotational Motion Sensor  reference=foundation.enum.MeasurementReference.difference  acceleration_port=false  velocity_port=true  position_port=true  wrap_angle=simscape.enum.onoff.off  offset=0 rad
  Measurement Filter : TransferFcn  Denominator=[0.001 1]
  Mechanical Rotational Reference2 : fl_lib/Mechanical/Rotational Elements/Mechanical Rotational Reference
  PS-Simulink Converter : nesl_utility/PS-Simulink Converter  PhysicalDomain=network_engine_domain  SubClassName=ps_output  LeftPortType=input  RightPortType=output  PseudoPeriodic=off  Frequencies=[]  VectorFormat=1-D array  Unit=rpm  AffineConversion=off
  R : PMIOPort  Side=Left
  wTurbine : Outport
  tag scope: wTurbine=global
  wires:
  PS-Simulink Converter/1 -> Measurement Filter/1
  Measurement Filter/1 -> [wTurbine], wTurbine/1
  connections:
  Ideal Rotational Motion Sensor/RConn2 -- PS-Simulink Converter/LConn1
  Ideal Rotational Motion Sensor/LConn1 -- R/RConn1
  Ideal Rotational Motion Sensor/RConn1 -- Mechanical Rotational Reference2/LConn1

== system sscv_wind_turbine/Pitch Controller/Turbine State 0 : Park Brake and Turbine State 3 : Pitch Brake/Turbine State 0 an 3 ==
  note: Turbine State 0 & 3: Park & Pitch Brake
  pitchState : Inport
  Enable : EnablePort  StatesWhenEnabling=reset
  Constant : Constant  Value=pitchBrakeAngle
  Constant1 : Constant
  Controller : TransferFcn  Denominator="[controllerTimeConstant  1]"
  Integrator : Integrator
  Switch : Switch  Criteria=u2 > Threshold  Threshold=controllerTimeConstant*log(1-(maxPitchAngle/pitchBrakeAngle))*(-1.01)  SaturateOnIntegerOverflow=off  InputSameDT=off
  pitchAngle : Outport
  wires:
  Integrator/1 -> Switch/2
  pitchState/1 -> Switch/3
  Constant1/1 -> Integrator/1
  Constant/1 -> Controller/1
  Controller/1 -> Switch/1
  Switch/1 -> pitchAngle/1

== system sscv_wind_turbine/Pitch Controller/Turbine State 1 : Startup Condition/Turbine State 1 ==
  note: Turbine State 1: Startup
  Enable : EnablePort  StatesWhenEnabling=reset
  Constant : Constant  Value=minPitchAngle
  Saturation : Saturate  UpperLimit=maxPitchAngle  LowerLimit=minPitchAngle
  Transfer Fcn : TransferFcn  Denominator=[controllerTimeConstant 1]
  pitchAngle : Outport
  wires:
  Constant/1 -> Transfer Fcn/1
  Saturation/1 -> pitchAngle/1
  Transfer Fcn/1 -> Saturation/1

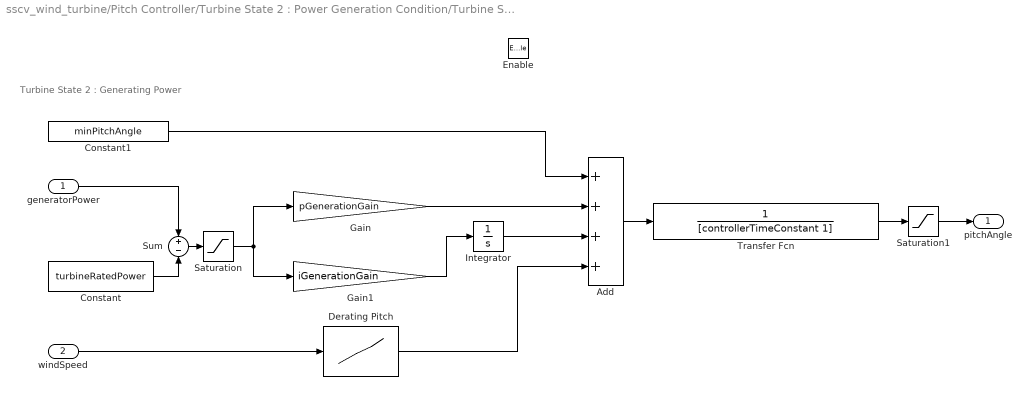
== system sscv_wind_turbine/Pitch Controller/Turbine State 2 : Power Generation Condition/Turbine State 2 ==
  note: Turbine State 2 : Generating Power
  generatorPower : Inport
  windSpeed : Inport  Port=2
  Enable : EnablePort  StatesWhenEnabling=reset
  Add : Sum  Inputs=++++
  Constant : Constant  Value=turbineRatedPower
  Constant1 : Constant  Value=minPitchAngle
  Derating Pitch : Lookup_n-D  NumberOfTableDimensions=1  BreakpointsForDimension1=Derating(:,1)  Table=Derating(:,2)-minPitchAngle  InternalRulePriority=Speed  RndMeth=Simplest
  Gain : Gain  Gain=pGenerationGain
  Gain1 : Gain  Gain=iGenerationGain
  Integrator : Integrator
  Saturation : Saturate  UpperLimit=inf  LowerLimit=0
  Saturation1 : Saturate  UpperLimit=maxPitchAngle  LowerLimit=minPitchAngle
  Sum : Sum  Inputs=+-
  Transfer Fcn : TransferFcn  Denominator=[controllerTimeConstant 1]
  pitchAngle : Outport
  wires:
  Saturation1/1 -> pitchAngle/1
  Gain/1 -> Add/2
  Constant1/1 -> Add/1
  Add/1 -> Transfer Fcn/1
  generatorPower/1 -> Sum/1
  Constant/1 -> Sum/2
  Sum/1 -> Saturation/1
  Saturation/1 -> Gain/1, Gain1/1
  Transfer Fcn/1 -> Saturation1/1
  Integrator/1 -> Add/3
  Gain1/1 -> Integrator/1
  windSpeed/1 -> Derating Pitch/1
  Derating Pitch/1 -> Add/4

== system sscv_wind_turbine/Wind Turbine/Nacelle/Brakes ==
  parkingBrake : Inport
  Disk Friction Clutch : sdl_lib/Clutches/Disc Friction Clutch  geometry_model=1  r_eff=brakeTorqueRadius m  d_o=150 mm  d_i=100 mm  nS=numFrictionSurfaces  piston_area=brakePistonArea m^2  unidirectional=0  enable_faults=simscape.enum.onoff.off  fault_type=sdl.enum.clutchFault.lock  friction_model=1  mu_w_vector=[1 1e8] rad/s  temperature_TLU=[280.0, 300.0, 320.0] K  mu_static=brakeStaticFrictionCoeff  mu_static_vector=[0.4, 0.38, 0.36]  mu_coulomb=brakeKineticFrictionCoeff  mu_coulomb_vector=[0.3 0.001]  mu_coulomb_temp_vector=[0.3, 0.28, 0.25]  mu_coulomb_matrix=[0.34, 0.32, 0.3; 0.3, 0.28, 0.25; 0.25, 0.2, 0.15]  mu_interp_method=1  mu_extrap_method=1  d_f=1  w_tol=brakeClutchVelocityTol rad/s  pressure_min=brakeThresholdPressure Pa  mu_visc=0 N*m/(rad/s)  initial_state_locked=sdl.enum.initial_lock.unlocked  thermal_mass=25 kJ/K  T_init=300 K
      settings: InternalSimscapePortConfiguration="{\"Bottom\":[],\"Left\":[{\"id\":\"P\",\"label\":\"P\",\"type\":\"input\"},{\"id\":\"B\",\"label\":\"B\",\"type\":\"foundation.mechanical.rotational.rotational\"}],\"Right\":[{\"id\":\"F\",\"label\":\"F\",\"type\":\"foundation.mechanical.rotational.rotational\"}],\"Top\":[]}"
  Engagement Pressure : Gain  Gain=brakePressure
  Mechanical Rotational Reference : fl_lib/Mechanical/Rotational Elements/Mechanical Rotational Reference
  Simulink-PS Converter : nesl_utility/Simulink-PS Converter  PhysicalDomain=network_engine_domain  SubClassName=ps_input  LeftPortType=input  RightPortType=output  PseudoPeriodic=off  Frequencies=[]  NoiseDistribution=none  NoiseParameters=[]  Unit=bar  AffineConversion=off  FilteringAndDerivatives=zero  SimscapeFilterOrder=1  InputFilterTimeConstant=0.005  UdotUserProvided=0
  R : PMIOPort  Tag=PMCPort  Side=Left
  wires:
  Engagement Pressure/1 -> Simulink-PS Converter/1
  parkingBrake/1 -> Engagement Pressure/1
  connections:
  Disk Friction Clutch/RConn1 -- Mechanical Rotational Reference/LConn1
  R/RConn1 -- Disk Friction Clutch/LConn2
  Simulink-PS Converter/RConn1 -- Disk Friction Clutch/LConn1

== system sscv_wind_turbine/Wind Turbine/Nacelle/Gear Tain ==
  Helical Gear First Step : sdl_lib/Gears/Simple Gear  ratio=firstStepTeethRatio  rotation_direction=sdl.enum.shaftOutputDirection.opposite  enable_faults=simscape.enum.onoff.off  efficiency_fault=0.05  fault_angles=pi / 12 rad  friction_model=sdl.enum.gear_efficiencies_load.constant  T_noload=0.1 N*m  T_nom=5 N*m  efficiency_nom=0.8  efficiency=0.95  temperature_TLU=[ 280 300 320 ] K  load_TLU=[ 1 5 10 ] N*m  efficiency_TLU=[ 0.95 0.9 0.85 ]  efficiency_TLU2=[ 0.85 0.8 0.75; 0.95 0.9 0.85; 0.85 0.8 0.7 ]  w_thr=0.01 rad/s  pwr_thr=0.001 W  enable_backlash=false  hardstop_model=simscape.enum.hardstop.smooth  backlash_distance=1e-3 mm  r_base=0.1 m  transition=1e-4 mm  backlash_stiffness=1e7 N/m  backlash_damping=1e6 N/(m/s)  coeff_rest=0  v_tol=0.001 m/s  f_tol=0 N  mu_visc=[ 0 0 ] N*m/(rad/s)  thermal_mass=50 J/K  temperature_specify=off  temperature_priority=High  temperature=300 K  temperature_nominal_specify=off  temperature_nominal_value=1  temperature_nominal_unit=K  x_backlash_specify=off  x_backlash_priority=None  x_backlash=0 mm  x_backlash_nominal_specify=off  x_backlash_nominal_value=1  x_backlash_nominal_unit=mm  f_hardstop_specify=off  f_hardstop_priority=None  f_hardstop=0 N  f_hardstop_nominal_specify=off  f_hardstop_nominal_value=1  f_hardstop_nominal_unit=N  v_backlash_specify=off  v_backlash_priority=None  v_backlash=0 m/s  v_backlash_nominal_specify=off  v_backlash_nominal_value=1  v_backlash_nominal_unit=m/s
  Helical Gear Second Step : sdl_lib/Gears/Simple Gear  ratio=secondStepTeethRatio  rotation_direction=sdl.enum.shaftOutputDirection.same  enable_faults=simscape.enum.onoff.off  efficiency_fault=0.05  fault_angles=pi / 12 rad  friction_model=sdl.enum.gear_efficiencies_load.constant  T_noload=0.1 N*m  T_nom=5 N*m  efficiency_nom=0.8  efficiency=0.95  temperature_TLU=[ 280 300 320 ] K  load_TLU=[ 1 5 10 ] N*m  efficiency_TLU=[ 0.95 0.9 0.85 ]  efficiency_TLU2=[ 0.85 0.8 0.75; 0.95 0.9 0.85; 0.85 0.8 0.7 ]  w_thr=0.01 rad/s  pwr_thr=0.001 W  enable_backlash=false  hardstop_model=simscape.enum.hardstop.smooth  backlash_distance=1e-3 mm  r_base=0.1 m  transition=1e-4 mm  backlash_stiffness=1e7 N/m  backlash_damping=1e6 N/(m/s)  coeff_rest=0  v_tol=0.001 m/s  f_tol=0 N  mu_visc=[ 0 0 ] N*m/(rad/s)  thermal_mass=50 J/K  temperature_specify=off  temperature_priority=High  temperature=300 K  temperature_nominal_specify=off  temperature_nominal_value=1  temperature_nominal_unit=K  x_backlash_specify=off  x_backlash_priority=None  x_backlash=0 mm  x_backlash_nominal_specify=off  x_backlash_nominal_value=1  x_backlash_nominal_unit=mm  f_hardstop_specify=off  f_hardstop_priority=None  f_hardstop=0 N  f_hardstop_nominal_specify=off  f_hardstop_nominal_value=1  f_hardstop_nominal_unit=N  v_backlash_specify=off  v_backlash_priority=None  v_backlash=0 m/s  v_backlash_nominal_specify=off  v_backlash_nominal_value=1  v_backlash_nominal_unit=m/s
  Inertia Carrier Shaft : fl_lib/Mechanical/Rotational Elements/Inertia  inertia=carrierShaftInertia kg*m^2  num_ports=foundation.enum.numPorts2.one  w_specify=on  w_priority=None  w=0 rad/s  w_nominal_specify=off  w_nominal_value=1  w_nominal_unit=rad/s  t_specify=off  t_priority=High  t=0 N*m  t_nominal_specify=off  t_nominal_value=1  t_nominal_unit=N*m
  Inertia First Step Shaft : fl_lib/Mechanical/Rotational Elements/Inertia  inertia=stepShaftInertia kg*m^2  num_ports=foundation.enum.numPorts2.one  w_specify=on  w_priority=None  w=0 rad/s  w_nominal_specify=off  w_nominal_value=1  w_nominal_unit=rad/s  t_specify=off  t_priority=High  t=0 N*m  t_nominal_specify=off  t_nominal_value=1  t_nominal_unit=N*m
  Mechanical Rotational Reference1 : fl_lib/Mechanical/Rotational Elements/Mechanical Rotational Reference
  Planetary Gear : sdl_lib/Gears/Planetary Gear  rs_ratio=ringSunTeethRatio  friction_model=sdl.enum.gear_friction.constant  efficiency=[ 0.95 0.95 ]  temperature_TLU=[ 280 300 320 ] K  efficiency_sp_TLU=[ 0.95 0.9 0.85 ]  efficiency_rp_TLU=[ 0.95 0.9 0.85 ]  pwr_thr=[ 0.001 0.001 ] W  mu_visc=[0 0] N*m/(rad/s)  model_inertia=simscape.enum.onoff.off  planet_inertia=0.001 kg*m^2  thermal_mass=50 J/K  T_init=300 K
  R : PMIOPort  Side=Left
  C : PMIOPort  Port=2  Side=Right
  connections:
  Helical Gear Second Step/LConn1 -- C/RConn1
  Planetary Gear/RConn2 -- Inertia Carrier Shaft/LConn1 -- Helical Gear First Step/RConn1
  R/RConn1 -- Planetary Gear/LConn1
  Mechanical Rotational Reference1/LConn1 -- Planetary Gear/RConn1
  Helical Gear Second Step/RConn1 -- Inertia First Step Shaft/LConn1 -- Helical Gear First Step/LConn1

== system sscv_wind_turbine/Wind Turbine/Nacelle/Generator Velocity Sensor  ==
  Ideal Rotational Motion Sensor : fl_lib/Mechanical/Mechanical Sensors/Ideal Rotational Motion Sensor  reference=foundation.enum.MeasurementReference.difference  acceleration_port=false  velocity_port=true  position_port=true  wrap_angle=simscape.enum.onoff.off  offset=0 rad
  Measurement Filter : TransferFcn  Denominator=[0.001 1]
  Mechanical Rotational Reference2 : fl_lib/Mechanical/Rotational Elements/Mechanical Rotational Reference
  PS-Simulink Converter : nesl_utility/PS-Simulink Converter  PhysicalDomain=network_engine_domain  SubClassName=ps_output  LeftPortType=input  RightPortType=output  PseudoPeriodic=off  Frequencies=[]  VectorFormat=1-D array  Unit=rpm  AffineConversion=off
  R : PMIOPort  Side=Left
  wGen : Outport
  wires:
  Measurement Filter/1 -> wGen/1
  PS-Simulink Converter/1 -> Measurement Filter/1
  connections:
  Ideal Rotational Motion Sensor/RConn2 -- PS-Simulink Converter/LConn1
  Ideal Rotational Motion Sensor/LConn1 -- R/RConn1
  Ideal Rotational Motion Sensor/RConn1 -- Mechanical Rotational Reference2/LConn1
